simulink model "echo_model"  (R2022b)
settings: Solver=VariableStepAuto  StartTime=0.0  StopTime=10.0  RelTol=1e-3
settings Model: Creator=berka  LastModifiedBy=berka

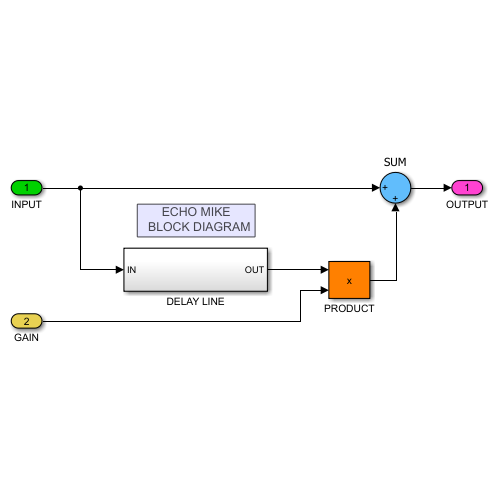
[thumbnail: Simulink's stored preview of the top-level diagram]
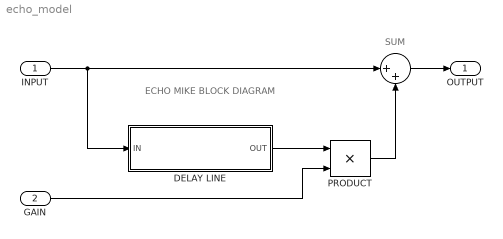
== system echo_model ==
  note: ECHO MIKE
      |   BLOCK DIAGRAM
  note: SUM
  INPUT : Inport
  GAIN : Inport  Port=2
  " " : Sum  Inputs=|++
  DELAY LINE : Subsystem
  PRODUCT : Product
  OUTPUT : Outport
  wires:
  GAIN/1 -> PRODUCT/2
  DELAY LINE/1(OUT) -> PRODUCT/1
  " "/1 -> OUTPUT/1
  PRODUCT/1 -> " "/2
  INPUT/1 -> DELAY LINE/1("IN "), " "/1

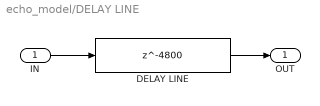
== system echo_model/DELAY LINE ==
  "IN " : Inport
  DELAY LINE : Delay  DelayLength=4800  InitialCondition=0
  OUT : Outport
  wires:
  "IN "/1 -> DELAY LINE/1
  DELAY LINE/1 -> OUT/1
